simulink model "constantVeltoLeader"  (R2019a)
settings: Solver=VariableStepAuto  StartTime=0.0  StopTime=inf  RelTol=1e-3
undefined symbols (not defined in the file or in its folder): Angular, Linear
libraries: robotlib x2
settings Model: Creator=ruby  LastModifiedBy=ruby

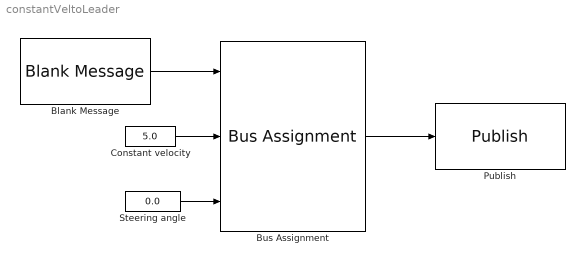
== system constantVeltoLeader ==
  Blank Message : robotlib/Blank Message  messageClass=Message  entityType=geometry_msgs/Twist  messageType=geometry_msgs/Twist  SampleTime=inf
      settings: SourceProductBaseCode=RO
  Bus Assignment : BusAssignment  AssignedSignals=Linear.X,Angular.Z
  Constant velocity : Constant  Value=5.0
  Publish : robotlib/Publish  topicSource=Select from ROS network  topic=/leadVehicle/cmd_vel  messageType=geometry_msgs/Twist  messageQueueLength=1
      settings: SourceProductBaseCode=RO
  Steering angle : Constant  Value=0.0
  wires:
  Bus Assignment/1 -> Publish/1
  Blank Message/1 -> Bus Assignment/1
  Constant velocity/1 -> Bus Assignment/2
  Steering angle/1 -> Bus Assignment/3
